simulink model "trajectory_planner"  (R2025b)
settings: configuration reference "MCConfiguration" (kept outside this file)
libraries: simulink x1, arsenal x1, dspsigops x1
settings Model: DataDictionary=embeddedBoard_common.sldd  Creator=rpumpo  LastModifiedBy=mfussi
settings ConfigSetRef: SourceName=MCConfiguration

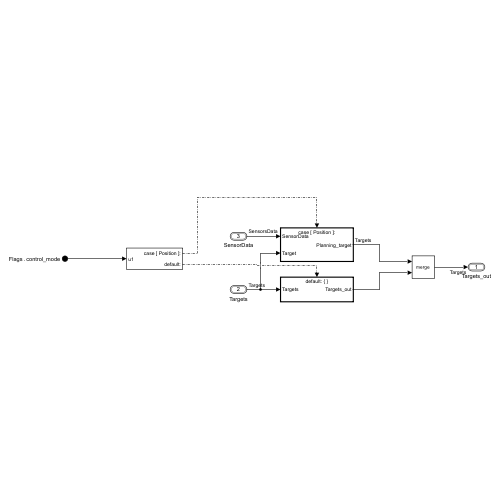
[thumbnail: Simulink's stored preview of the top-level diagram]
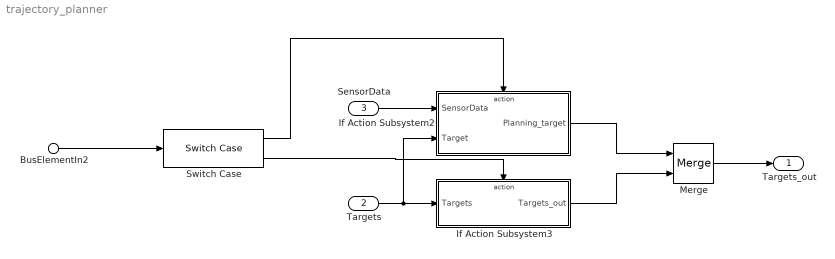
== system trajectory_planner ==
  BusElementIn2 : Inport  Description=control mode  PortName=Flags  Element=control_mode
  Targets : Inport  Port=2  OutDataTypeStr=Bus: Targets  BusOutputAsStruct=on
  SensorData : Inport  Port=3  OutDataTypeStr=Bus: SensorsData  BusOutputAsStruct=on
  If Action Subsystem2 : Subsystem  TreatAsAtomicUnit=on
  If Action Subsystem3 : Subsystem  TreatAsAtomicUnit=on
  Merge : Merge
  Switch Case : SwitchCase  CaseConditions={ControlModes.Position}
  Targets_out : Outport  OutDataTypeStr=Bus: Targets  BusOutputAsStruct=on
  wires:
  BusElementIn2/1 -> Switch Case/1
  Targets/1 -> If Action Subsystem2/2(Target), If Action Subsystem3/1(Targets)
  If Action Subsystem2/1(Planning_target) -> Merge/1
  SensorData/1 -> If Action Subsystem2/1(SensorData)
  Switch Case/1 -> If Action Subsystem2/Action
  Switch Case/2 -> If Action Subsystem3/Action
  Merge/1 -> Targets_out/1
  If Action Subsystem3/1(Targets_out) -> Merge/2

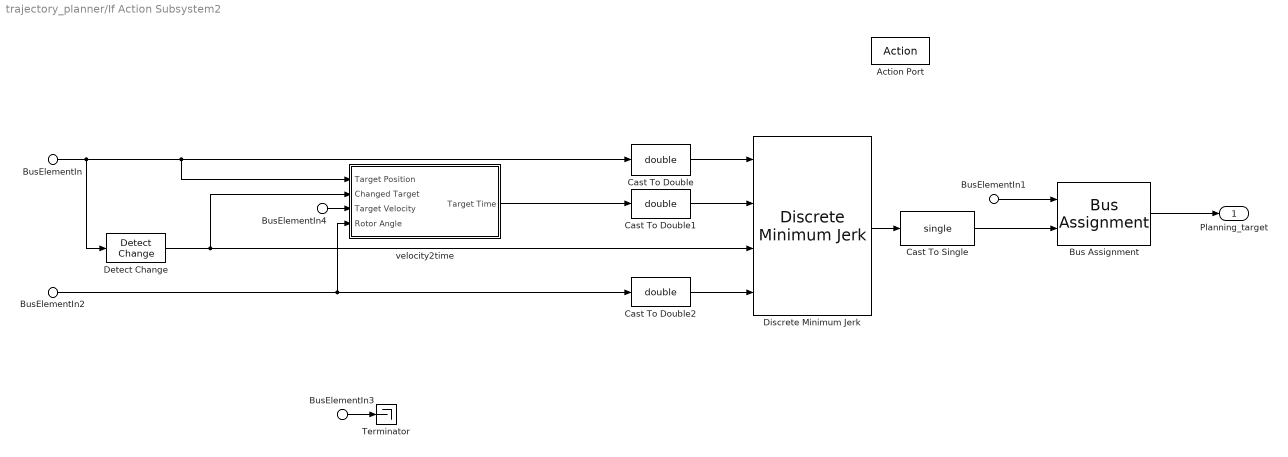
== system trajectory_planner/If Action Subsystem2 ==
  BusElementIn2 : Inport  Description=Mechanical Angle before gearbox  PortName=SensorData  Element=motorsensors.qencoder.rotor_angle
  BusElementIn1 : Inport  Port=2  PortName=Target
  BusElementIn3 : Inport  Description=Target time for position control  Port=2  PortName=Target  Element=trajectory_time
  BusElementIn : Inport  Port=2  PortName=Target  Element=position
  BusElementIn4 : Inport  Port=2  PortName=Target  Element=velocity
  Action Port : ActionPort  ActionPortLabel=case [ Position ]:
  Bus Assignment : BusAssignment  AssignedSignals=position
  Cast To Double : DataTypeConversion  OutDataTypeStr=double  SaturateOnIntegerOverflow=off  RndMeth=Floor
  Cast To Double1 : DataTypeConversion  OutDataTypeStr=double  SaturateOnIntegerOverflow=off  RndMeth=Floor
  Cast To Double2 : DataTypeConversion  OutDataTypeStr=double  SaturateOnIntegerOverflow=off  RndMeth=Floor
  Cast To Single : DataTypeConversion  OutDataTypeStr=single  SaturateOnIntegerOverflow=off  RndMeth=Floor
  Detect Change : simulink/Logic and Bit Operations/Detect Change  vinit=0  OutDataTypeStr=boolean
  Discrete Minimum Jerk : arsenal/Filters/Discrete Minimum Jerk  Ts=0.001
      settings: SourceProductName=iCub Tech Arsenal
  Terminator : Terminator
  velocity2time : Subsystem
  Planning_target : Outport  OutDataTypeStr=Bus: Targets  BusOutputAsStruct=on
  wires:
  Bus Assignment/1 -> Planning_target/1
  BusElementIn1/1 -> Bus Assignment/1
  Cast To Double1/1 -> Discrete Minimum Jerk/2
  Cast To Double/1 -> Discrete Minimum Jerk/1
  BusElementIn2/1 -> Cast To Double2/1, velocity2time/4(Rotor Angle)
  Cast To Double2/1 -> Discrete Minimum Jerk/4
  BusElementIn/1 -> Cast To Double/1, velocity2time/1(Target Position), Detect Change/1
  Discrete Minimum Jerk/1 -> Cast To Single/1
  Cast To Single/1 -> Bus Assignment/2
  Detect Change/1 -> velocity2time/2(Changed Target), Discrete Minimum Jerk/3
  BusElementIn3/1 -> Terminator/1
  BusElementIn4/1 -> velocity2time/3(Target Velocity)
  velocity2time/1(Target Time) -> Cast To Double1/1

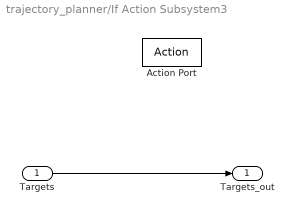
== system trajectory_planner/If Action Subsystem3 ==
  Targets : Inport  OutDataTypeStr=Bus: Targets
  Action Port : ActionPort  ActionPortLabel=default:
  Targets_out : Outport  OutDataTypeStr=Bus: Targets
  wires:
  Targets/1 -> Targets_out/1

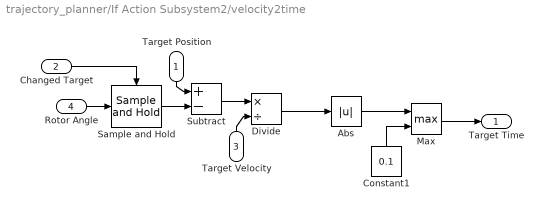
== system trajectory_planner/If Action Subsystem2/velocity2time ==
  Target Position : Inport
  Changed Target : Inport  Port=2
  Target Velocity : Inport  Port=3
  Rotor Angle : Inport  Port=4
  Abs : Abs  SaturateOnIntegerOverflow=off
  Constant1 : Constant  Value=0.1  OutDataTypeStr=single
  Divide : Product  Inputs=*/
  Max : MinMax  Function=max  Inputs=2
  Sample and Hold : dspsigops/Sample and Hold  trig=Rising edge  initCond=0  latchinput=off
  Subtract : Sum  Inputs=+-
  Target Time : Outport
  wires:
  Divide/1 -> Abs/1
  Target Velocity/1 -> Divide/2
  Subtract/1 -> Divide/1
  Constant1/1 -> Max/2
  Abs/1 -> Max/1
  Sample and Hold/1 -> Subtract/2
  Max/1 -> Target Time/1
  Changed Target/1 -> Sample and Hold/Trigger
  Target Position/1 -> Subtract/1
  Rotor Angle/1 -> Sample and Hold/1
